simulink library "AR_Drone_Actuators"  (R2016a)
settings: Solver=ode45  StartTime=0.0  StopTime=10.0  RelTol=1e-3
libraries: simulink x5
settings Model: Creator=sannem  LastModifiedBy=sannem
settings DataIOCC: LimitDataPoints=on
settings DebuggingCC: AllowSymbolicDim=off

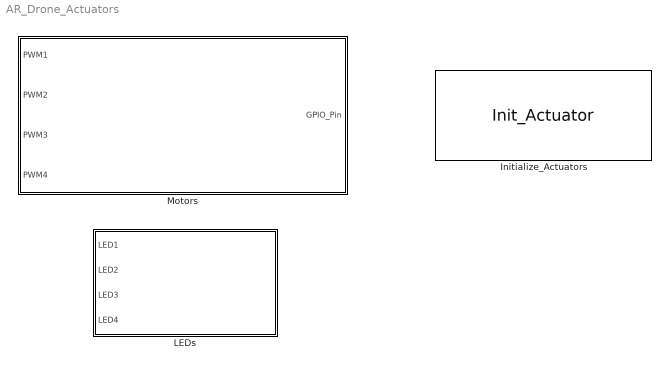
== system AR_Drone_Actuators ==
  Initialize_Actuators : S-Function  FunctionName=Init_Actuator  SFunctionDeploymentMode=off  EnableBusSupport=off  mask{SFunctionSpec=, ShowSpec=on}
      mask prompts: ShowSpec "Display function specification"
      mask help: This block must be placed in the Simulink model to be able to use the motor actuator and LED blocks
      mask Callback ShowSpec:
      | if strcmp(get_param(gcbh, 'ShowSpec'), 'on')
      |   set_param(gcbh, 'MaskDisplay', sprintf('fprintf(''%s'');', get_param(gcbh, 'SFunctionSpec')));
      | else
      |   set_param(gcbh, 'MaskDisplay', sprintf('fprintf(''%s'');', get_param(gcbh, 'FunctionName')));
      | end
      mask Display: fprintf('');
  LEDs : Subsystem
      mask help:
      | The quadcopter has 4 LEDs, one for each of the motors. The LEDs can emit 3 colours viz. RED, GREEN AND ORANGE. The input to the block are integers from 0-3 and the numbers represent the colours as follows:
      |
      | 0 - OFF
      | 1 - RED
      | 2 - GREEN
      | 3 - ORANGE
      settings: CopyFcn=%check_init_block  DeleteFcn=%clear x  DestroyFcn=%clear x
      mask Display:
      | fprintf('LED Color Input')
      | port_label('input',1,'LED1');
      | port_label('input',2,'LED2');
      | port_label('input',3,'LED3');
      | port_label('input',4,'LED4');
  Motors : Subsystem
      mask help: The quadcopter has 4 rotors. The input to the rotors are PWM values which are percentage of the full speed of the rotor with 0% being no speed and 100% being full speed. The inputs values are limited to this range. The block converts the 4 PWM values into a 40 bit number which is then fed to the motor controller.
      settings: CopyFcn=%check_init_block
      mask Display:
      | fprintf('Propeller Actuation Input');
      | port_label('input',1,'PWM1');
      | port_label('input',2,'PWM2');
      | port_label('input',3,'PWM3');
      | port_label('input',4,'PWM4');
      | port_label('output',1,'GPIO_Fault_Pin');

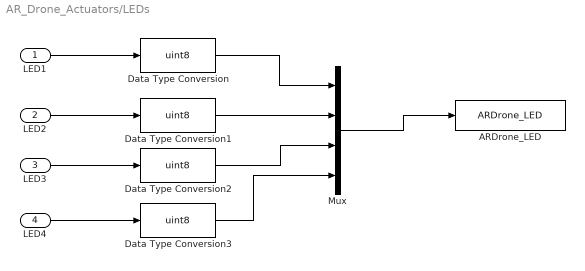
== system AR_Drone_Actuators/LEDs ==
  LED1 : Inport
  LED2 : Inport  Port=2
  LED3 : Inport  Port=3
  LED4 : Inport  Port=4
  ARDrone_LED : S-Function  FunctionName=ARDrone_LED  SFunctionDeploymentMode=off  EnableBusSupport=off  mask(Legacy Function){SFunctionSpec=LED_set(uint8 u1[4]), ShowSpec=on}
      mask prompts: ShowSpec "Display function specification"
      mask help:
      | This block allows you to call the legacy functions specified by the following Legacy Code Tool definition:
      | def.SFunctionName = 'ARDrone_LED';
      | def.OutputFcnSpec = 'LED_set(uint8 u1[4])';
      | def.HeaderFiles = {'led.h'};
      | def.SourceFiles = {'led.c'};
      | def.IncPaths = {'.'};
      mask Help: <p>This block was generated automatically by the Legacy Code Tool. For detailed help on this tool, call<a href="matlab:legacy_code('help')"> legacy_code('help')</a>.</p>
      mask Callback ShowSpec:
      | if strcmp(get_param(gcbh, 'ShowSpec'), 'on')
      |   set_param(gcbh, 'MaskDisplay', sprintf('fprintf(''%s'');', get_param(gcbh, 'SFunctionSpec')));
      | else
      |   set_param(gcbh, 'MaskDisplay', sprintf('fprintf(''%s'');', get_param(gcbh, 'FunctionName')));
      | end
      mask Display: fprintf('LED_set(uint8 u1[4])');
  Data Type Conversion{,1..3} (4 alike) : DataTypeConversion  OutDataTypeStr=uint8
  Mux : Mux
  wires:
  LED2/1 -> Data Type Conversion1/1
  LED1/1 -> Data Type Conversion/1
  Mux/1 -> ARDrone_LED/1
  LED4/1 -> Data Type Conversion3/1
  Data Type Conversion/1 -> Mux/1
  Data Type Conversion1/1 -> Mux/2
  Data Type Conversion3/1 -> Mux/4
  LED3/1 -> Data Type Conversion2/1
  Data Type Conversion2/1 -> Mux/3

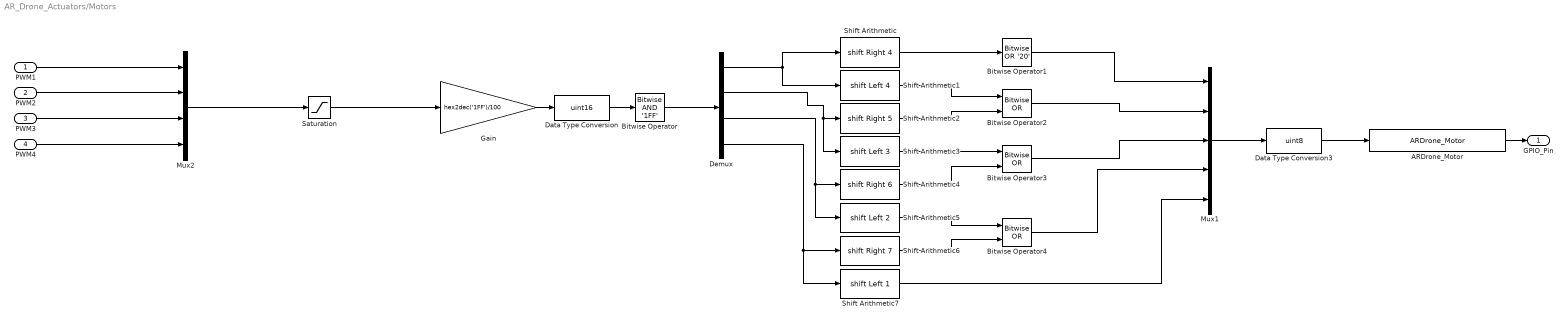
== system AR_Drone_Actuators/Motors ==
  PWM1 : Inport
  PWM2 : Inport  Port=2
  PWM3 : Inport  Port=3
  PWM4 : Inport  Port=4
  ARDrone_Motor : S-Function  FunctionName=ARDrone_Motor  SFunctionDeploymentMode=off  EnableBusSupport=off  mask(Legacy Function){SFunctionSpec=uint16 y1 = Motor_Set(uint8 u1[5]), ShowSpec=on}
      mask prompts: ShowSpec "Display function specification"
      mask help:
      | This block allows you to call the legacy functions specified by the following Legacy Code Tool definition:
      | def.SFunctionName = 'ARDrone_Motor';
      | def.OutputFcnSpec = 'uint16 y1 = Motor_Set(uint8 u1[5])';
      | def.HeaderFiles = {'motor.h'};
      | def.SourceFiles = {'motor.c'};
      | def.IncPaths = {'.'};
      mask Help: <p>This block was generated automatically by the Legacy Code Tool. For detailed help on this tool, call<a href="matlab:legacy_code('help')"> legacy_code('help')</a>.</p>
      mask Callback ShowSpec:
      | if strcmp(get_param(gcbh, 'ShowSpec'), 'on')
      |   set_param(gcbh, 'MaskDisplay', sprintf('fprintf(''%s'');', get_param(gcbh, 'SFunctionSpec')));
      | else
      |   set_param(gcbh, 'MaskDisplay', sprintf('fprintf(''%s'');', get_param(gcbh, 'FunctionName')));
      | end
      mask Display: fprintf('uint16 y1 = Motor_Set(uint8 u1[5])');
  Bitwise Operator : simulink/Logic and Bit Operations/Bitwise Operator  logicop=AND  UseBitMask=on  BitMask='1FF'  BitMaskRealWorld=Stored Integer
  Bitwise Operator1 : simulink/Logic and Bit Operations/Bitwise Operator  logicop=OR  UseBitMask=on  BitMask='20'  BitMaskRealWorld=Stored Integer
  Bitwise Operator2 : simulink/Logic and Bit Operations/Bitwise Operator  logicop=OR  UseBitMask=off  NumInputPorts=2  BitMask='20'  BitMaskRealWorld=Stored Integer
  Bitwise Operator3 : simulink/Logic and Bit Operations/Bitwise Operator  logicop=OR  UseBitMask=off  NumInputPorts=2  BitMask='20'  BitMaskRealWorld=Stored Integer
  Bitwise Operator4 : simulink/Logic and Bit Operations/Bitwise Operator  logicop=OR  UseBitMask=off  NumInputPorts=2  BitMask='20'  BitMaskRealWorld=Stored Integer
  Data Type Conversion : DataTypeConversion  OutDataTypeStr=uint16
  Data Type Conversion3 : DataTypeConversion  OutDataTypeStr=uint8
  Demux : Demux
  Gain : Gain  Gain=hex2dec('1FF')/100
  Mux1 : Mux  Inputs=5
  Mux2 : Mux
  Saturation : Saturate  UpperLimit=100  LowerLimit=0
  Shift Arithmetic : ArithShift  BitShiftNumber=4  BitShiftDirection=Right
  Shift Arithmetic1 : ArithShift  BitShiftNumber=4  BitShiftDirection=Left
  Shift Arithmetic2 : ArithShift  BitShiftNumber=5  BitShiftDirection=Right
  Shift Arithmetic3 : ArithShift  BitShiftNumber=3  BitShiftDirection=Left
  Shift Arithmetic4 : ArithShift  BitShiftNumber=6  BitShiftDirection=Right
  Shift Arithmetic5 : ArithShift  BitShiftNumber=2  BitShiftDirection=Left
  Shift Arithmetic6 : ArithShift  BitShiftNumber=7  BitShiftDirection=Right
  Shift Arithmetic7 : ArithShift  BitShiftNumber=1  BitShiftDirection=Left
  GPIO_Pin : Outport
  wires:
  Data Type Conversion/1 -> Bitwise Operator/1
  Mux1/1 -> Data Type Conversion3/1
  Shift Arithmetic3/1 -> Bitwise Operator3/1
  Shift Arithmetic2/1 -> Bitwise Operator2/2
  Bitwise Operator3/1 -> Mux1/3
  Shift Arithmetic6/1 -> Bitwise Operator4/2
  PWM1/1 -> Mux2/1
  Gain/1 -> Data Type Conversion/1
  Bitwise Operator1/1 -> Mux1/1
  Demux/4 -> Shift Arithmetic7/1, Shift Arithmetic6/1
  Bitwise Operator2/1 -> Mux1/2
  Data Type Conversion3/1 -> ARDrone_Motor/1
  Shift Arithmetic5/1 -> Bitwise Operator4/1
  Demux/2 -> Shift Arithmetic3/1, Shift Arithmetic2/1
  Shift Arithmetic7/1 -> Mux1/5
  PWM4/1 -> Mux2/4
  PWM2/1 -> Mux2/2
  PWM3/1 -> Mux2/3
  Bitwise Operator4/1 -> Mux1/4
  Mux2/1 -> Saturation/1
  Shift Arithmetic/1 -> Bitwise Operator1/1
  Saturation/1 -> Gain/1
  Shift Arithmetic1/1 -> Bitwise Operator2/1
  Bitwise Operator/1 -> Demux/1
  Demux/3 -> Shift Arithmetic5/1, Shift Arithmetic4/1
  Shift Arithmetic4/1 -> Bitwise Operator3/2
  Demux/1 -> Shift Arithmetic/1, Shift Arithmetic1/1
  ARDrone_Motor/1 -> GPIO_Pin/1
